simulink model "controller_template"  (Simulink 7.8)
settings: Solver=FixedStepDiscrete  SolverMode=SingleTasking  StartTime=0.0  StopTime=inf  FixedStep=Ts  RelTol=1e-3
PreLoadFcn:
  | load_waypoints
  | main;
StopFcn:
  | y_ref_wall = RecordYZ.signals(1).values(:,2);
  | y_wall = RecordYZ.signals(1).values(:,1);
  | 
  | z_ref_wall = RecordYZ.signals(2).values(:,2);
  | z_wall = RecordYZ.signals(2).values(:,1);
  | 
  | close all;
  | figure;
  | plot(y_ref_wall,z_ref_wall,'b','LineWidth',2); hold on;
  | plot(y_wall,z_wall,'r','LineWidth',2); grid on;
  | plot(traj_FG.X_ref_y_real(1,:),-traj_FG.X_ref_z_real(1,:),'o-g');
  | axis equal;
values from neighbouring files (symbols this model uses):
  Add_pitch = [0.764669359834 -6.55628329998 0 0 0.0133529191446 -0.0326334422872 0 0 0 0 0 0 ... (16 elements, 4x4)]    [kostas_malakies.mat]    (also in kostas_malakies2.mat)
  Aff_pitch = [0.764669359834 -6.55628329998 -0.0099932514458 -0.411590904828 0.0133529191446 -0.0326334422872 -8.8646944178e-05 -0.00470014240893 0 0 1 0 ... (16 elements, 4x4)]    [kostas_malakies.mat]    (also in kostas_malakies2.mat)
  Aff_roll = [0.825180563081 -6.10606264808 -0.00763580464276 -0.367448917026 0.0145694646817 0.0253169520582 -6.457583527e-05 -0.00409059128644 0 0 1 0 ... (16 elements, 4x4)]    [kostas_malakies.mat]    (also in kostas_malakies2.mat; main.m = [Aff_roll,zeros(size(Aff_roll,1),1);zeros(1,size(Aff_roll,1); main_last.m = [Aff_roll,zeros(size(Aff_roll,1),1);zeros(1,size(Aff_roll,1))
  Bdd_pitch = [0.235330640166  -0.000506747889746; 6.55628329998  -0.0141179351932; 0  0; 0  0]    [kostas_malakies.mat]    (also in kostas_malakies2.mat)
  Bff_pitch = [0.235330640166  0; 6.55628329998  0; -0.000567656018985  0; -0.0435256495914  0]    [kostas_malakies.mat]    (also in kostas_malakies2.mat)
  Bff_roll = [0.174819436919  0; 6.10606264808  0; -0.000299760068643  0; -0.0270637325616  0]    [kostas_malakies.mat]    (also in kostas_malakies2.mat; main.m = [Bff_roll;zeros(1,size(Bff_roll,2))]; main_last.m = [Bff_roll;zeros(1,size(Bff_roll,2))])
  Fi_Xdir = [-3.0499319419 0 -7.4272134917 -0.3906339295 0 0 -7.4272134917 -1.4749060606 -2.0114272215 -3.0499319419 -7.4272134917 -1.154776828 ... (624 elements, 156x4)]    [kostas_malakies.mat]    (also in kostas_malakies2.mat = [0 0 -2.6412818692 0 0 -3.3089352882 0 -2.6412818692 0 -2.64)
  Fi_XdirFF = [-0.447351940284 0 0 -1.28434394361 -4.04417159595 -1.80654990505 -1.28434394361 1 -4.04417159595 -1.80654990505 1 0 ... (536 elements, 134x4)]    [kostas_malakies.mat]    (also in kostas_malakies2.mat; matlab.mat = [-1.62441280603 -1.28434394361 -1.7723315065 -1.66810627541 )
  Fi_Yaw = [-1.14619813144 0 0]    [kostas_malakies.mat]    (also in kostas_malakies2.mat; matlab.mat = -0.284754025426)
  Fi_Ydir = [-0.466308586531 2.22044604925e-16 2.22044604925e-16 -1.46518332723 -4.54395337171 -2.00318743375 -1.46518332723 1 -4.54395337171 -2.00318743375 1 2.22044604925e-16 ... (536 elements, 134x4)]    [kostas_malakies.mat]    (also in kostas_malakies2.mat = [-0.521298425559 -2.64128186917 -15.6565978667 -8.2066553194; matlab.mat = [1 -1.9173235349 -1.46518332723 1 1 1 1 1 -1.98764774833 -1.)
  Fi_Zdir = [0 -1.80359099426e-16 0 1.4149586889 0 0 2.30859647265e-14 -5.77149118162e-15 0 0 0 0 ... (54 elements, 27x2)]    [kostas_malakies.mat]    (also in kostas_malakies2.mat = [4.30976351396 0 4.73307471514 3.80948040666 0 0 0 0.5468933; matlab.mat = [0 -9.51943523339e-14 0 1.99761158231 0 1.18992940417e-14 0 )
  g = 9.8065    [kostas_malakies.mat]    (also in kostas_malakies2.mat; load_PMModel.m = 9.81; main.m; main_last.m)
  Gi_Xdir = [33.5705355246 -0.267 268.54680224 -0.0188924328 -0.267 -0.267 268.54680224 0.039239647 0.0672163769 0.1708155012 1.343002558 0.0122735546 ... (156 elements, 156x1)]    [kostas_malakies.mat]    (also in kostas_malakies2.mat = [-0.267 -0.267 -1.8623973597 -0.267 -0.267 16.4050483477 -0.)
  Gi_XdirFF = [0 0.27 -0.27 0.478341621792 -6.42962779272 -1.98615606962 -0.478341621792 -0.373552567526 6.42962779272 1.98615606962 0.373552567526 0.27 ... (134 elements, 134x1)]    [kostas_malakies.mat]    (also in kostas_malakies2.mat; matlab.mat = [3.88578058619e-16 0.478341621792 -0.139455879222 -0.1159311)
  Gi_Yaw = [4.4408920985e-16 -3.14159265359 3.14159265359]    [kostas_malakies.mat]    (also in kostas_malakies2.mat = [-4.4408920985e-16 -3.14159265359 3.14159265359]; matlab.mat = 4.4408920985e-16)
  Gi_Ydir = [-2.77555756156e-16 0.27 -0.27 0.516209388722 7.06668201156 2.10835273651 -0.516209388722 -0.383863816771 -7.06668201156 -2.10835273651 0.383863816771 0.27 ... (134 elements, 134x1)]    [kostas_malakies.mat]    (also in kostas_malakies2.mat = [1.11022302463e-16 0.765579126644 531.260413192 11.754237275; matlab.mat = [0.383863816771 -0.133207088705 0.516209388722 0.38386381677)
  Gi_Zdir = [-1 -1 -1 2.22044604925e-16 -1 -1 -1 -1 1 -1 -1 -1 ... (27 elements, 27x1)]    [kostas_malakies.mat]    (also in kostas_malakies2.mat = [0.174387892495 -1 0.368373831608 3.33066907388e-16 -1 -1 -1; matlab.mat = [-2 -2 -2 1.11022302463e-15 -2 -2 -2 2 -2 -2 -2 2 ... (21 el)
  Hn_Xdir = [0.0894044100374 0.0185803675847 -0.0787469077295 -1 0 0.0903062437314 0.0275585020049 -0.0791302456941 -0.0894044100374 -0.0892208721324 -1 0 ... (5248 elements, 1312x4)]    [kostas_malakies.mat]    (also in kostas_malakies2.mat = [0.194772943522 -0.999280166414 0.0919386851603 -0.143548982)
  Hn_XdirFF = [-0.618529611748 0.618529611748 0.827215259158 -0.512155371354 -0.650909395739 -0.827215259158 0.930717154057 0.512155371354 0.650909395739 -0.930717154057 -1 0 ... (4464 elements, 1116x4)]    [kostas_malakies.mat]    (also in kostas_malakies2.mat; matlab.mat = [1 -0.136019433325 -0.405248495598 -0.339279056031 0 -1 0.13)
  Hn_Yaw = [1 -1 -1 1 1 -1]    [kostas_malakies.mat]    (also in kostas_malakies2.mat; matlab.mat = [1 -1])
  Hn_Ydir = [-0.642151612842 0.642151612842 0.873369621238 0.521434628645 0.668917219747 -0.873369621238 0.934789012395 -0.521434628645 -0.668917219747 -0.934789012395 -1 0 ... (4532 elements, 1133x4)]    [kostas_malakies.mat]    (also in kostas_malakies2.mat = [0.972602710123 0.0284063109089 0.559530157965 0.73050130567; matlab.mat = [0.711566553558 0.999813894311 -0.735660470031 0 0 0.5471922)
  Hn_Zdir = [-0.560552458797 -0.996815278536 -0.988320507921 0.666673243042 -1 0 -0.421994354267 -0.987440631917 -0.973284290019 -0.956170964903 -0.936236606521 0.560552458797 ... (224 elements, 112x2)]    [kostas_malakies.mat]    (also in kostas_malakies2.mat = [-0.781813705838 -0.712499731132 0.751798766698 0 -0.7286973; matlab.mat = [1 -1 -0.996815278536 -0.990718937584 -0.276007160242 0.3840)
  kalm_mpc_yaw =     [kostas_malakies.mat]    (also in kostas_malakies2.mat)
  Kn_Xdir = [0.991899150003 0.997410232697 -0.994647298545 0.5094 5 0.992251952723 0.997427328059 -0.992171068824 -0.991899150003 -0.991948411946 0.5094 5 ... (1312 elements, 1312x1)]    [kostas_malakies.mat]    (also in kostas_malakies2.mat = [0.972973501195 0.603589097273 0.988510480824 -0.97816203365)
  Kn_XdirFF = [0.373314565409 0.373314565409 0.472754204418 0.915522246067 0.951154784392 0.472754204418 0.240212330437 0.915522246067 0.951154784392 0.240212330437 0.2094 2 ... (1116 elements, 1116x1)]    [kostas_malakies.mat]    (also in kostas_malakies2.mat; matlab.mat = [0.2094 0.19132523886 0.382063154155 0.900203176458 2 0.2094)
  Kn_Yaw = [2.74088097634 2.74088097634 -2.74088097634 3.14159265359 -2.74088097634 3.14159265359]    [kostas_malakies.mat]    (also in kostas_malakies2.mat; matlab.mat = [0.0873 0.0873])
  Kn_Ydir = [0.371815875743 0.371815875743 0.451349483511 0.90366201682 0.917647772499 0.451349483511 0.24471770913 0.90366201682 0.917647772499 0.24471770913 0.2094 2 ... (1133 elements, 1133x1)]    [kostas_malakies.mat]    (also in kostas_malakies2.mat = [0.351231202126 0.997082913977 0.855763802521 0.792250278627; matlab.mat = [-0.126119149197 0.0536759032179 0.37354703421 2 2 -0.239682)
  Kn_Zdir = [0.727672356179 1.00172267683 1.00656919451 -0.471160923828 1 1 1.18526984431 1.00688561667 1.01272393898 1.01603878926 1.01572683497 -0.727672356179 ... (112 elements, 112x1)]    [kostas_malakies.mat]    (also in kostas_malakies2.mat = [0.21304012328 0.326509029469 -0.262060822346 1 0.301409884 ; matlab.mat = [1 1 1.00663007512 1.02122194908 0.632590992205 -0.384463644)
  MAX_BIAS_YAW_RATE = 0.0872664625997    [kostas_malakies.mat]    (also in kostas_malakies2.mat; main.m; main_last.m)
  Nc_Xdir = [5 10 5 15 8 13 7 11 8 9 8 8 ... (156 elements, 156x1)]    [kostas_malakies.mat]    (also in kostas_malakies2.mat = [11 10 8 9 9 7 13 7 10 7 6 12 ... (277 elements, 277x1)])
  Nc_XdirFF = [18 15 15 11 9 7 11 14 9 7 14 8 ... (134 elements, 134x1)]    [kostas_malakies.mat]    (also in kostas_malakies2.mat; matlab.mat = [14 8 7 10 8 7 10 12 10 10 12 11 ... (107 elements, 107x1)])
  Nc_Yaw = [2 2 2]    [kostas_malakies.mat]    (also in kostas_malakies2.mat; matlab.mat = 2)
  Nc_Ydir = [18 16 16 10 9 7 10 14 9 7 14 8 ... (134 elements, 134x1)]    [kostas_malakies.mat]    (also in kostas_malakies2.mat = [22 12 6 9 9 5 12 13 6 9 9 5 ... (171 elements, 171x1)]; matlab.mat = [11 8 12 15 7 9 10 13 10 14 12 7 ... (104 elements, 104x1)])
  Nc_Zdir = [6 7 3 6 3 4 4 3 6 5 3 4 ... (27 elements, 27x1)]    [kostas_malakies.mat]    (also in kostas_malakies2.mat = [4 4 3 12 5 4 3 3 4 3 3 4 ... (93 elements, 93x1)]; matlab.mat = [6 3 7 4 4 3 4 6 3 5 3 3 ... (21 elements, 21x1)])
  pitch_cmd2pitch_1stOrd = 1.42468924998    [kostas_malakies.mat]    (also in kostas_malakies2.mat)
  roll_cmd2roll_1stOrd = 1.38101661575    [kostas_malakies.mat]    (also in kostas_malakies2.mat)
  thrust_cmd2thrust_0thOrd = 0.876575459522    [kostas_malakies.mat]    (also in kostas_malakies2.mat)
  THRUST_CMD_GAIN = -0.0835    [kostas_malakies.mat]    (also in kostas_malakies2.mat; load_PMModel.m)
  traj_FG =     [kostas.mat]    (also in kostas_malakies.mat; kostas_malakies2.mat; main.m = ReferenceCreator(maxdisty,maxdistz,scale_y,scale_z); main_last.m = ReferenceCreator(maxdisty,maxdistz,scale_y,scale_z))
  Ts = 0.02    [kostas_malakies.mat]    (also in kostas_malakies2.mat; main.m; main_last.m; matlab.mat = 0.08)
  yaw_cmd2yaw_1stOrd = 2.01792090263    [kostas_malakies.mat]    (also in kostas_malakies2.mat)
  z = [-0.93079906702 -0.933865725994 -0.937557637691 -0.939011216164 -0.94143640995 -0.944628417492 -0.947235524654 -0.949601888657 -0.952827751637 -0.9567258358 -0.958320975304 -0.960991024971 ... (7988 elements, 7988x1)]    [kostas_malakies2.mat]    (also in plotDataTest.m = simout_data.signals.values(:,11))
libraries: simulink x48, Hquad_control_LIB_MPC x13
(part 3 of 3)

== system controller_template/FreeFlight Pos Ctrl/MAIN CONTROL LOOP1/x controller MPC FG  /Explicit Ctrl Hybrid/PitchPropagate ==
  uprev : Inport
  x : Inport  Port=2
  Constant : Constant  Value=Aff_pitch
  Constant1 : Constant  Value=Bff_pitch
  Constant2 : Constant  Value=Add_pitch
  Constant3 : Constant  Value=Bdd_pitch
  Demux : Demux
  Demux1 : Demux
  MATLAB Function : MATLAB Function  TreatAsAtomicUnit=on
  Mux : Mux
  Mux1 : Mux
  Saturation : Saturate  UpperLimit=0.2094  LowerLimit=-0.2094
  Saturation1 : Saturate  UpperLimit=2  LowerLimit=-2
  Saturation2 : Saturate  UpperLimit=1  LowerLimit=-1
  Saturation3 : Saturate  UpperLimit=0  LowerLimit=-1
  Switch : Switch  Criteria=u2 ~= 0
  Switch1 : Switch  Criteria=u2 ~= 0
  Out1 : Outport
  wires:
  uprev/1 -> MATLAB Function/4(u)
  x/1 -> Demux1/1
  Mux/1 -> Out1/1
  Saturation/1 -> Mux/1
  Saturation1/1 -> Mux/2
  Saturation2/1 -> Mux/4
  Saturation3/1 -> Mux/3
  MATLAB Function/1(y) -> Demux/1
  Constant2/1 -> Switch/3
  Constant/1 -> Switch/1
  Switch/1 -> MATLAB Function/2(A)
  Constant1/1 -> Switch1/1
  Constant3/1 -> Switch1/3
  Switch1/1 -> MATLAB Function/3(B)
  Demux1/1 -> Mux1/1
  Demux1/2 -> Mux1/2
  Demux1/3 -> Mux1/3, Switch/2, Switch1/2
  Demux1/4 -> Mux1/4
  Mux1/1 -> MATLAB Function/1(x)
  Demux/1 -> Saturation/1
  Demux/2 -> Saturation1/1
  Demux/3 -> Saturation3/1
  Demux/4 -> Saturation2/1

== system controller_template/FreeFlight Pos Ctrl/MAIN CONTROL LOOP1/y controller MPC FG/Explicit Ctrl1/RollPropagate ==
  uprev : Inport
  x : Inport  Port=2
  Constant : Constant  Value=Aff_roll
  Constant1 : Constant  Value=Bff_roll
  MATLAB Function : MATLAB Function  TreatAsAtomicUnit=on
  Out1 : Outport
  wires:
  MATLAB Function/1(y) -> Out1/1
  x/1 -> MATLAB Function/1(x)
  uprev/1 -> MATLAB Function/4(u)
  Constant/1 -> MATLAB Function/2(A)
  Constant1/1 -> MATLAB Function/3(B)

== system controller_template/FreeFlight Pos Ctrl/MAIN CONTROL LOOP1/yaw controller MPC FG/Explicit Ctrl1/YawPropagate ==
  uprev : Inport
  x : Inport  Port=2
  Constant : Constant
  Constant1 : Constant  Value=0
  MATLAB Function : MATLAB Function  TreatAsAtomicUnit=on
  Out1 : Outport
  wires:
  MATLAB Function/1(y) -> Out1/1
  x/1 -> MATLAB Function/1(x)
  uprev/1 -> MATLAB Function/4(u)
  Constant1/1 -> MATLAB Function/3(B)
  Constant/1 -> MATLAB Function/2(A)

== matlab function FreeFlight Pos Ctrl/MAIN CONTROL LOOP1/x controller MPC FG /Explicit Ctrl Hybrid/Ctrl_Xdir ==
  data: X input double; U output double; Hn input double; Kn input double; Fi input double; Gi input double; Nc input double; flag_oob output double
function [U,flag_oob] = OptimalMPCInput(X,Hn,Kn,Fi,Gi,Nc)

tolerance = 1;
nr  = size(Nc,1);
MPT_ABSTOL = 1e-8;
minreg = 0;
X = round(10000*X)/10000;

flag_oob = 0;
%maxSize = max(Nc);

Hi = zeros(1000,4);
Ki = zeros(1000,1);

% Find the proper region
abspos = 1;
for ireg = 1:nr
    sumViol = 0;
    isinside = 1;
    

  %  Hi(1:Nc(ireg),1:4) = Hn(abspos:(abspos+Nc(ireg)-1),1:4);
    for i = 1:Nc(ireg)
        for j = 1:4
            Hi(i,j) = Hn(abspos + i - 1,j);
        end
    end
    
%    Ki(1:Nc(ireg),1) = Kn(abspos:(abspos+Nc(ireg)-1),1);
    for i = 1:Nc(ireg)
        Ki(i,1) = Kn(abspos + i - 1,1);
    end
    abspos = abspos + Nc(ireg);
    
    F = Fi(ireg,:);
    G = Gi(ireg,:);
    
    nc = Nc(ireg);
    
    for ic = 1:nc
        hx = Hi(ic,:)*X;
        if ((hx - Ki(ic)) > MPT_ABSTOL)
            isinside = 0;
            sumViol = sumViol + (hx - Ki(ic));
        end
    end
    
    if (sumViol < tolerance)
        tolerance = sumViol;
        minreg = ireg;
    end
    % extract the right control law
    if (isinside == 1)
        U = F*X + G;
        return
    end
end
F = Fi(minreg,:);
G = Gi(minreg,:);
U = F*X + G;
flag_oob = 1;
return

== matlab function FreeFlight Pos Ctrl/MAIN CONTROL LOOP1/y controller MPC FG/Explicit Ctrl1/Ctrl_Xdir ==
  data: X input double; U output double; Hn input double; Kn input double; Fi input double; Gi input double; Nc input double; flag_oob output double
function [U,flag_oob] = OptimalMPCInput(X,Hn,Kn,Fi,Gi,Nc)

tolerance = 1;
nr  = size(Nc,1);
MPT_ABSTOL = 1e-8;
minreg = 0;
X = round(10000*X)/10000;

flag_oob = 0;
%maxSize = max(Nc);

Hi = zeros(100,5);
Ki = zeros(100,1);

% Find the proper region
abspos = 1;
for ireg = 1:nr
    sumViol = 0;
    isinside = 1;
    

  %  Hi(1:Nc(ireg),1:4) = Hn(abspos:(abspos+Nc(ireg)-1),1:4);
    for i = 1:Nc(ireg)
        for j = 1:5
            Hi(i,j) = Hn(abspos + i - 1,j);
        end
    end
    
%    Ki(1:Nc(ireg),1) = Kn(abspos:(abspos+Nc(ireg)-1),1);
    for i = 1:Nc(ireg)
        Ki(i,1) = Kn(abspos + i - 1,1);
    end
    abspos = abspos + Nc(ireg);
    
    F = Fi(ireg,:);
    G = Gi(ireg,:);
    
    nc = Nc(ireg);
    
    for ic = 1:nc
        hx = Hi(ic,:)*X;
        if ((hx - Ki(ic)) > MPT_ABSTOL)
            isinside = 0;
            sumViol = sumViol + (hx - Ki(ic));
        end
    end
    
    if (sumViol < tolerance)
        tolerance = sumViol;
        minreg = ireg;
    end
    % extract the right control law
    if (isinside == 1)
        U = F*X + G;
        return
    end
end
F = Fi(minreg,:);
G = Gi(minreg,:);
U = F*X + G;
flag_oob = 1;
%U = U_prev;
return

== matlab function FreeFlight Pos Ctrl/MAIN CONTROL LOOP1/z controller MPC FG/Explicit Ctrl1/Ctrl_Xdir ==
  data: X input double; U output double; Hn input double; Kn input double; Fi input double; Gi input double; Nc input double; flag_oob output double
function [U,flag_oob] = OptimalMPCInput(X,Hn,Kn,Fi,Gi,Nc)

tolerance = 1;
nr  = size(Nc,1);
MPT_ABSTOL = 1e-8;
minreg = 0;
X = round(10000*X)/10000;

flag_oob = 0;
%maxSize = max(Nc);

Hi = zeros(100,3);
Ki = zeros(100,1);

% Find the proper region
abspos = 1;
for ireg = 1:nr
    sumViol = 0;
    isinside = 1;
    

  %  Hi(1:Nc(ireg),1:4) = Hn(abspos:(abspos+Nc(ireg)-1),1:4);
    for i = 1:Nc(ireg)
        for j = 1:3
            Hi(i,j) = Hn(abspos + i - 1,j);
        end
    end
    
%    Ki(1:Nc(ireg),1) = Kn(abspos:(abspos+Nc(ireg)-1),1);
    for i = 1:Nc(ireg)
        Ki(i,1) = Kn(abspos + i - 1,1);
    end
    abspos = abspos + Nc(ireg);
    
    F = Fi(ireg,:);
    G = Gi(ireg,:);
    
    nc = Nc(ireg);
    
    for ic = 1:nc
        hx = Hi(ic,:)*X;
        if ((hx - Ki(ic)) > MPT_ABSTOL)
            isinside = 0;
            sumViol = sumViol + (hx - Ki(ic));
        end
    end
    
    if (sumViol < tolerance)
        tolerance = sumViol;
        minreg = ireg;
    end
    % extract the right control law
    if (isinside == 1)
        U = F*X + G;
        return
    end
end
F = Fi(minreg,:);
G = Gi(minreg,:);
U = F*X + G;
flag_oob = 1;
%U = U_prev;
return

== matlab function FreeFlight Pos Ctrl/MAIN CONTROL LOOP1/yaw controller MPC FG/Explicit Ctrl1/Ctrl_Xdir ==
  data: X input double; U output double; Hn input double; Kn input double; Fi input double; Gi input double; Nc input double; flag_oob output double
function [U,flag_oob] = OptimalMPCInput(X,Hn,Kn,Fi,Gi,Nc)

tolerance = 1;
nr  = size(Nc,1);
MPT_ABSTOL = 1e-8;
minreg = 0;
X = round(10000*X)/10000;

flag_oob = 0;
%maxSize = max(Nc);

Hi = zeros(100,1);
Ki = zeros(100,1);

% Find the proper region
abspos = 1;
for ireg = 1:nr
    sumViol = 0;
    isinside = 1;
    

  %  Hi(1:Nc(ireg),1:4) = Hn(abspos:(abspos+Nc(ireg)-1),1:4);
    for i = 1:Nc(ireg)
        for j = 1:1
            Hi(i,j) = Hn(abspos + i - 1,j);
        end
    end
    
%    Ki(1:Nc(ireg),1) = Kn(abspos:(abspos+Nc(ireg)-1),1);
    for i = 1:Nc(ireg)
        Ki(i,1) = Kn(abspos + i - 1,1);
    end
    abspos = abspos + Nc(ireg);
    
    F = Fi(ireg,:);
    G = Gi(ireg,:);
    
    nc = Nc(ireg);
    
    for ic = 1:nc
        hx = Hi(ic,:)*X;
        if ((hx - Ki(ic)) > MPT_ABSTOL)
            isinside = 0;
            sumViol = sumViol + (hx - Ki(ic));
        end
    end
    
    if (sumViol < tolerance)
        tolerance = sumViol;
        minreg = ireg;
    end
    % extract the right control law
    if (isinside == 1)
        U = F*X + G;
        return
    end
end
F = Fi(minreg,:);
G = Gi(minreg,:);
U = F*X + G;
flag_oob = 1;
%U = U_prev;
return

== matlab function FreeFlight Pos Ctrl/MAIN CONTROL LOOP1/y controller MPC FG/Explicit Ctrl1/RollPropagate/MATLAB Function ==
  data: x input double; y output double; A input double; B input double; u input double
function y = fcn(x,A,B,u)
%#codegen

y = A*x + B*[u;0];

== matlab function FreeFlight Pos Ctrl/MAIN CONTROL LOOP1/yaw controller MPC FG/Explicit Ctrl1/YawPropagate/MATLAB Function ==
  data: x input double; y output double; A input double; B input double; u input double
function y = fcn(x,A,B,u)
%#codegen

y = A*x + B*u;

== matlab function FreeFlight Pos Ctrl/MAIN CONTROL LOOP1/x controller MPC FG /Explicit Ctrl Hybrid/PitchPropagate/MATLAB Function ==
  data: x input double; y output double; A input double; B input double; u input double
function y = fcn(x,A,B,u)
%#codegen

y = A*x + B*[u;0];

== matlab function FreeFlight Pos Ctrl/Subsystem/Wall Point Reference/Wall Deviation/MATLAB Function ==
  data: u input double; y output double; thres input double
function y = fcn(u,thres)
%#codegen
if u >=thres
    y = 0;
else
    y = u;
end

== matlab function FreeFlight Pos Ctrl/decoupling and rotation/decoupling /Embedded MATLAB Function ==
  data: pitch_cmd_comp output double; roll_cmd_comp output double; pitch_meas input double; thrust_comp output double; roll_meas input double; pitch_cmd input double; roll_cmd input double; thrust input double; m input double; g input double; posx input double
function [pitch_cmd_comp, roll_cmd_comp, thrust_comp]  = fcn(pitch_meas, roll_meas, pitch_cmd, roll_cmd, thrust,m,g,posx)
%#eml
maxangle = 4*pi/180;
thrust_comp=thrust;
if (posx == 0)
    thrust_comp=thrust/(cos(pitch_meas)*cos(roll_meas));
    
    if abs(pitch_meas) >= maxangle && abs(roll_meas) >= maxangle
        thrust_comp=thrust/(cos(maxangle)*cos(maxangle));
    elseif abs(pitch_meas) >= maxangle
        thrust_comp=thrust/(cos(maxangle)*cos(roll_meas));
    elseif abs(roll_meas) >= maxangle
        thrust_comp=thrust/(cos(pitch_meas)*cos(maxangle));
    end
else
    thrust_comp=thrust/(cos(pitch_meas)*cos(roll_meas));
end
pitch_cmd_comp = m*g/thrust_comp*pitch_cmd;
roll_cmd_comp = m*g/thrust_comp*roll_cmd;

% pitch_cmd_comp=pitch_cmd;
% roll_cmd_comp=roll_cmd;
% pitch_cmd_comp = atan(Fx/(-thrust_comp));
% roll_cmd_comp = atan(Fy/(thrust_comp));

% pitch_cmd_comp = atan(-g*m*pitch_cmd/(-thrust));
% roll_cmd_comp = atan(g*m*roll_cmd*cos(pitch_meas)/(thrust));

== matlab function FreeFlight Pos Ctrl/decoupling and rotation/rotate_to_quat_frame/Embedded MATLAB Function ==
  data: yaw input double; pitch_rot output double; pitch_cmd input double; roll_cmd input double; pitch_bias input double; roll_bias input double; roll_rot output double; pitch_bias_rot output double; roll_bias_rot output double
function [pitch_rot,roll_rot, pitch_bias_rot,roll_bias_rot] = fcn(yaw, pitch_cmd, roll_cmd, pitch_bias, roll_bias)

sin_yaw=sin(yaw);
cos_yaw=cos(yaw);

R=[cos_yaw, sin_yaw; -sin_yaw, cos_yaw];

temp=R'*[pitch_cmd;roll_cmd];
pitch_rot=temp(1);
roll_rot=temp(2);

temp=R'*[pitch_bias;roll_bias];
pitch_bias_rot=temp(1);
roll_bias_rot=temp(2);

== matlab function FreeFlight Pos Ctrl/Subsystem/Wall Point Reference/Subsystem/MATLAB Function ==
  data: en_flag input double; count_out output double; en_flag_prev input double; count_out_prev input double
function count_out = fcn(en_flag,en_flag_prev,count_out_prev)
%#codegen

count_out = count_out_prev; 
if( ((en_flag == 1) && (en_flag_prev == 0)) || ((en_flag == 1) && (en_flag_prev == 1)) )
    count_out = count_out_prev + 1;
end

end

== matlab function FreeFlight Pos Ctrl/MAIN CONTROL LOOP1/Subsystem/MATLAB Function ==
  data: pitch_cmd input double; pitch_cmd_out output double; pitch_angle input double; dist_wall input double; K_gain input double; max_neg_pitch input double; additive_pitch input double; ratio_free_flight input double
function pitch_cmd_out = fcn(pitch_cmd,pitch_angle,dist_wall,K_gain,max_neg_pitch,additive_pitch,ratio_free_flight)
%#codegen

pitch_cmd_out = pitch_cmd;
ratio_free_flight = min(ratio_free_flight,1);

pitch_cmd_out = pitch_cmd_out + ratio_free_flight*additive_pitch;

if( (dist_wall == 0) && (pitch_angle < -max_neg_pitch) )
    pitch_cmd_out = pitch_cmd_out + K_gain*abs(pitch_angle + max_neg_pitch);
    pitch_cmd_out = pitch_cmd_out + (1-ratio_free_flight)*additive_pitch;
end

end

== matlab function FreeFlight Pos Ctrl/MAIN CONTROL LOOP1/y controller MPC FG/Wall Deviation/MATLAB Function ==
  data: u input double; y output double; thres input double
function y = fcn(u,thres)
%#codegen
if u >=thres
    y = 0.1;
else
    y = u;
end

== matlab function FreeFlight Pos Ctrl/MAIN CONTROL LOOP1/z controller MPC FG/Wall Deviation/MATLAB Function ==
  data: u input double; y output double; thres input double
function y = fcn(u,thres)
%#codegen
if u >=thres
    y = 0.1;
else
    y = u;
end

== matlab function FreeFlight Pos Ctrl/MAIN CONTROL LOOP1/x controller MPC FG /Wall Deviation/MATLAB Function ==
  data: u input double; y output double; thres input double
function y = fcn(u,thres)
%#codegen
if u >=thres
    y = 0;
else
    y = u;
end

== matlab function FreeFlight Pos Ctrl/MAIN CONTROL LOOP1/z controller MPC FG/Subsystem/MATLAB Function ==
  data: u_thrust input double; u_thrust_out output double; dx input double; dz input double; K_g_up input double
function u_thrust_out = fcn(u_thrust,dx,dz,K_g_up)
%#codegen

u_thrust_out = u_thrust;

if( dx>0 && dz<0 )
    u_thrust_out = K_g_up*u_thrust;
end

end

== matlab function FreeFlight Pos Ctrl/MAIN CONTROL LOOP1/y controller MPC FG/Subsystem/MATLAB Function ==
  data: input input double; input_out output double; dist_wall input double; K_gain input double
function input_out = fcn(input,dist_wall,K_gain)
%#codegen

input_out = input;

if(dist_wall>=0)
    input_out = input*K_gain;
end

end

== matlab function FreeFlight Pos Ctrl/Subsystem/Wall Point Reference/Subsystem1/MATLAB Function ==
  data: nominal_window_z input double; nominal_window_z_out output double; nominal_window_y input double; vel_z input double; vel_y input double; thres_vel_z input double; thres_vel_y input double; K_gain input double; maxDeltaWindow input double; nominal_window_y_out output double
function [nominal_window_z_out,nominal_window_y_out] = fcn(nominal_window_z,nominal_window_y,vel_z,vel_y,thres_vel_z,thres_vel_y,K_gain,maxDeltaWindow)
%#codegen

nominal_window_z_out = nominal_window_z;
nominal_window_y_out = nominal_window_y;

vel_y = abs(vel_y);
vel_z = (vel_z);

if( vel_y > thres_vel_y )
    nominal_window_y_out = nominal_window_y - min(K_gain*abs(vel_y - thres_vel_y),maxDeltaWindow);
end

if( vel_z > thres_vel_z )
    nominal_window_z_out = nominal_window_z - min(K_gain*abs(vel_z - thres_vel_z),maxDeltaWindow);
end

end

== matlab function FreeFlight Pos Ctrl/Free Flight Reference/create traj/generate_X_ref_x ==
  data: traj_x input double; X_ref_x output double; idx input double
function X_ref_x  = fcn(traj_x,idx)

pred_horizon_x=30;

X_ref_x=traj_x(:,idx:idx+pred_horizon_x);

== matlab function FreeFlight Pos Ctrl/Free Flight Reference/create traj/generate_X_ref_y ==
  data: traj_y input double; X_ref_y output double; idx input double
function X_ref_y  = fcn(traj_y,idx)

pred_horizon_y=30;

X_ref_y=traj_y(:,idx:idx+pred_horizon_y);

== matlab function FreeFlight Pos Ctrl/Free Flight Reference/create traj/generate_X_ref_yaw ==
  data: X_ref_yaw_unbounded input double; X_ref_yaw output double; yaw_meas input double; idx input double
function X_ref_yaw  = fcn(X_ref_yaw_unbounded,yaw_meas,idx)

pred_horizon_yaw=30;

yaw0=X_ref_yaw_unbounded(1,idx);
yaw_diff=yaw_meas-yaw0;


yaw_offset=round(yaw_diff/(2*pi))*2*pi;

X_ref_yaw=[X_ref_yaw_unbounded(1,idx:idx+pred_horizon_yaw)+yaw_offset;...
    X_ref_yaw_unbounded(2,idx:idx+pred_horizon_yaw)];

== matlab function FreeFlight Pos Ctrl/Free Flight Reference/create traj/generate_X_ref_z ==
  data: traj_z input double; X_ref_z output double; idx input double
function X_ref_z  = fcn(traj_z,idx)

pred_horizon_z=30;

X_ref_z=traj_z(:,idx:idx+pred_horizon_z);

== matlab function FreeFlight Pos Ctrl/decoupling and rotation/decoupling /Wall Deviation/MATLAB Function ==
  data: u input double; y output double; thres input double
function y = fcn(u,thres)
%#codegen
if u >=thres
    y = 0;
else
    y = u;
end

== matlab function FreeFlight Pos Ctrl/MAIN CONTROL LOOP1/x controller MPC FG /Explicit Ctrl Free Flight/Ctrl_Xdir ==
  data: X input double; U output double; Hn input double; Kn input double; Fi input double; Gi input double; Nc input double; flag_oob output double
function [U,flag_oob] = OptimalMPCInput(X,Hn,Kn,Fi,Gi,Nc)

tolerance = 1;
nr  = size(Nc,1);
MPT_ABSTOL = 1e-8;
minreg = 0;
X = round(10000*X)/10000;

flag_oob = 0;
%maxSize = max(Nc);

Hi = zeros(1000,4);
Ki = zeros(1000,1);

% Find the proper region
abspos = 1;
for ireg = 1:nr
    sumViol = 0;
    isinside = 1;
    

  %  Hi(1:Nc(ireg),1:4) = Hn(abspos:(abspos+Nc(ireg)-1),1:4);
    for i = 1:Nc(ireg)
        for j = 1:4
            Hi(i,j) = Hn(abspos + i - 1,j);
        end
    end
    
%    Ki(1:Nc(ireg),1) = Kn(abspos:(abspos+Nc(ireg)-1),1);
    for i = 1:Nc(ireg)
        Ki(i,1) = Kn(abspos + i - 1,1);
    end
    abspos = abspos + Nc(ireg);
    
    F = Fi(ireg,:);
    G = Gi(ireg,:);
    
    nc = Nc(ireg);
    
    for ic = 1:nc
        hx = Hi(ic,:)*X;
        if ((hx - Ki(ic)) > MPT_ABSTOL)
            isinside = 0;
            sumViol = sumViol + (hx - Ki(ic));
        end
    end
    
    if (sumViol < tolerance)
        tolerance = sumViol;
        minreg = ireg;
    end
    % extract the right control law
    if (isinside == 1)
        U = F*X + G;
        return
    end
end
F = Fi(minreg,:);
G = Gi(minreg,:);
U = F*X + G;
flag_oob = 1;
return

== matlab function FreeFlight Pos Ctrl/MAIN CONTROL LOOP1/yaw controller MPC FG/MATLAB Function ==
  data: psi_meas input double; psi_prime output double; psi_prev input double
function psi_prime = fcn(psi_meas,psi_prev)
%#codegen

psi_prime = psi_meas;
% 
% if((abs(psi_meas - psi_prev)>= (pi-0.1))&&(psi_prev > 0))
%     psi_prime = pi + abs(pi - abs(psi_meas));
% end
% 
% if((abs(psi_meas - psi_prev)>= (pi-0.1))&&(psi_prev < 0))
%     psi_prime = -pi - abs(pi - abs(psi_meas));
% end


% if((psi_meas>=((45)/180)*pi)&&(psi_meas<=(pi)))
%     psi_prime = (psi_meas - pi) -(180/180)*pi;
% end


end

== matlab function FreeFlight Pos Ctrl/MAIN CONTROL LOOP1/x controller MPC FG /Explicit Ctrl Free Flight/PitchPropagateFF/MATLAB Function ==
  data: x input double; y output double; A input double; B input double; u input double
function y = fcn(x,A,B,u)
%#codegen

y = A*x + B*[u;0];

== matlab function FreeFlight Pos Ctrl/MAIN CONTROL LOOP1/yaw states estimator bias/discrete kalman filter ==
  data: A input double; B input double; state_est output double; C input double; D input double; Q input double; R input double; u input double; y input double; P input double; state input double; P_est output double
function [state_est,P_est]  = fcn(A,B,C,D,Q,R, u, y, P, state)
%#eml

% Kalman filter according to Welch & Bishop, An Introduction to the Kalman
% Filter

n=size(A,1);

% Time update
x_=A*state+B*u;
P_=A*P*A'+Q;
  
% Measurement update
K=P_*C'*(C*P_*C'+R)^-1;
state_est=x_+K*(y-C*x_);
P_est=(eye(n)-K*C)*P_;

== matlab function FreeFlight Pos Ctrl/MAIN CONTROL LOOP1/yaw states estimator bias/MATLAB Function ==
  data: psi_meas input double; psi_prime output double
function psi_prime = fcn(psi_meas)
%#codegen

psi_prime = psi_meas;


if((psi_meas>=((45)/180)*pi)&&(psi_meas<=(pi+0.0175*6.5)))
    psi_prime = (psi_meas - pi) -(180/180)*pi;
end

% if(psi_meas<=pi


end

== matlab function pos controller/MAIN CONTROL LOOP1/yaw states estimator bias/discrete kalman filter ==
  data: A input double; B input double; state_est output double; C input double; D input double; Q input double; R input double; u input double; y input double; P input double; state input double; P_est output double
function [state_est,P_est]  = fcn(A,B,C,D,Q,R, u, y, P, state)
%#eml

% Kalman filter according to Welch & Bishop, An Introduction to the Kalman
% Filter

n=size(A,1);

% Time update
x_=A*state+B*u;
P_=A*P*A'+Q;
  
% Measurement update
K=P_*C'*(C*P_*C'+R)^-1;
state_est=x_+K*(y-C*x_);
P_est=(eye(n)-K*C)*P_;

== matlab function FreeFlight Pos Ctrl/MAIN CONTROL LOOP1/yaw controller MPC FG/MATLAB Function1 ==
  data: psi_meas input double; psi_out output double; x_pos input double; x_w input double; thres_x input double; ref_yaw input double; delta_x output double
function [psi_out,delta_x] = fcn(psi_meas,x_pos,x_w,thres_x,ref_yaw)
%#codegen

psi_out = psi_meas;

if(x_w - x_pos<=thres_x)
    psi_out = ref_yaw;
end

delta_x = x_w - x_pos;

end

== matlab function FreeFlight Pos Ctrl/Subsystem/Wall Point Reference/create traj1/generate_X_ref_x ==
  data: traj_x input double; X_ref_x output double; idx input double
function X_ref_x  = fcn(traj_x,idx)

pred_horizon_x=30;

X_ref_x=traj_x(:,idx:idx+pred_horizon_x);

== matlab function FreeFlight Pos Ctrl/Subsystem/Wall Point Reference/create traj1/generate_X_ref_y ==
  data: traj_y input double; X_ref_y output double; idx input double
function X_ref_y  = fcn(traj_y,idx)

pred_horizon_y=30;

X_ref_y=traj_y(:,idx:idx+pred_horizon_y);

== matlab function FreeFlight Pos Ctrl/Subsystem/Wall Point Reference/create traj1/generate_X_ref_yaw ==
  data: X_ref_yaw_unbounded input double; X_ref_yaw output double; yaw_meas input double; idx input double
function X_ref_yaw  = fcn(X_ref_yaw_unbounded,yaw_meas,idx)

pred_horizon_yaw=30;

yaw0=X_ref_yaw_unbounded(1,idx);
yaw_diff=yaw_meas-yaw0;


yaw_offset=round(yaw_diff/(2*pi))*2*pi;

X_ref_yaw=[X_ref_yaw_unbounded(1,idx:idx+pred_horizon_yaw)+yaw_offset;...
    X_ref_yaw_unbounded(2,idx:idx+pred_horizon_yaw)];

== matlab function FreeFlight Pos Ctrl/Subsystem/Wall Point Reference/create traj1/generate_X_ref_z ==
  data: traj_z input double; X_ref_z output double; idx input double
function X_ref_z  = fcn(traj_z,idx)

pred_horizon_z=30;

X_ref_z=traj_z(:,idx:idx+pred_horizon_z);

== matlab function FreeFlight Pos Ctrl/Subsystem/Wall Point Reference/Next Ref ==
  data: dx input double; y input double; z input double; yref input double; zref input double; thresy input double; thresz input double; threszdown input double; en output double; numSamples input double; counter input double
function en = fcn(dx,y,z,yref,zref,thresy,thresz,threszdown,numSamples,counter)

if abs(y-yref) > thresy
    dy = 1;
else
    dy = 0; % in position
end

% if abs(z-zref) > thresz
%     dz = 1;
% else
%     dz = 0; % in position
% end



if ( (z-zref) > thresz || -(z - zref) > threszdown ) 
    dz = 1;
else
    dz = 0; % in position
end


if dy ~= 0 || dz ~= 0 || dx ~=0
    en = 0; % not yet in position, don't change reference
else
    if counter < numSamples
        en = 1; % in position, both deviations < thres, change ref. point.
    else
        en = 0;
    end
end

== matlab function FreeFlight Pos Ctrl/Free Flight Reference/create traj1/generate_X_ref_x ==
  data: traj_x input double; X_ref_x output double; idx input double
function X_ref_x  = fcn(traj_x,idx)

pred_horizon_x=30;

X_ref_x=traj_x(:,idx:idx+pred_horizon_x);

== matlab function FreeFlight Pos Ctrl/Free Flight Reference/create traj1/generate_X_ref_y ==
  data: traj_y input double; X_ref_y output double; idx input double
function X_ref_y  = fcn(traj_y,idx)

pred_horizon_y=30;

X_ref_y=traj_y(:,idx:idx+pred_horizon_y);

== matlab function FreeFlight Pos Ctrl/Free Flight Reference/create traj1/generate_X_ref_yaw ==
  data: X_ref_yaw_unbounded input double; X_ref_yaw output double; yaw_meas input double; idx input double
function X_ref_yaw  = fcn(X_ref_yaw_unbounded,yaw_meas,idx)

pred_horizon_yaw=30;

yaw0=X_ref_yaw_unbounded(1,idx);
yaw_diff=yaw_meas-yaw0;


yaw_offset=round(yaw_diff/(2*pi))*2*pi;

X_ref_yaw=[X_ref_yaw_unbounded(1,idx:idx+pred_horizon_yaw)+yaw_offset;...
    X_ref_yaw_unbounded(2,idx:idx+pred_horizon_yaw)];

== matlab function FreeFlight Pos Ctrl/Free Flight Reference/create traj1/generate_X_ref_z ==
  data: traj_z input double; X_ref_z output double; idx input double
function X_ref_z  = fcn(traj_z,idx)

pred_horizon_z=30;

X_ref_z=traj_z(:,idx:idx+pred_horizon_z);
